simulink model "Vex2022Modle"  (R2022b)
settings: Solver=FixedStepAuto  StartTime=0.0  StopTime=inf  RelTol=1e-3  EnableMultiTasking=on
libraries: vexarmcortexlib x16, RoboticsPlayground x1
settings Model: Creator=carol  LastModifiedBy=carol
settings DataIOCC: LimitDataPoints=on  SignalLoggingSaveFormat=ModelDataLogs  ReturnWorkspaceOutputs=off
settings OptimizationCC: ExpressionDepthLimit=2147483647  LifeSpan=Inf  MaxStackSize=64  EfficientTunableParamExpr=on
settings DebuggingCC: UnderspecifiedInitializationDetection=Classic  MergeDetectMultiDrivingBlocksExec=none  InheritedTsInSrcMsg=none  FcnCallInpInsideContextMsg=warning  StateNameClashWarn=warning  SFUnexpectedBacktrackingDiag=warning  SFNoUnconditionalDefaultTransitionDiag=warning  SFExecutionAtInitializationDiag=none  SFMachineParentedDataDiag=warning  ArithmeticOperatorsInVariantConditions=warning
settings HardwareCC: ProdBitPerPointer=32  ProdBitPerSizeT=32  ProdBitPerPtrDiffT=32  ProdLargestAtomicInteger=Long  ProdLargestAtomicFloat=Double  ProdIntDivRoundTo=Undefined  ProdWordSize=32  ProdHWDeviceType=ARM Compatible->ARM Cortex
settings ModelReferenceCC: EnableRefExpFcnMdlSchedulingChecks=on  PropagateSignalLabelsOutOfModel=off
settings SFSimCC: MATLABDynamicMemAlloc=off  CustomCodeUndefinedFunction=UseInterfaceOnly
settings RTWCC: Description=Embedded Coder  SystemTargetFile=ert.tlc  HardwareBoard=ARM Cortex-based VEX Microcontroller  TemplateMakefile=ert_default_tmf  Toolchain=GNU Tools for VEX ARM Cortex
settings CodeAppCC: IgnoreCustomStorageClasses=off  CustomSymbolStrType=$N$R$M  StateflowObjectComments=on  InternalIdentifier=Classic
settings ERTTargetCC: CodeReplacementLibrary=GCC ARM Cortex-M3  MultiwordLength=2048  ConvertIfToSwitch=off  SuppressUnreachableDefaultCases=off

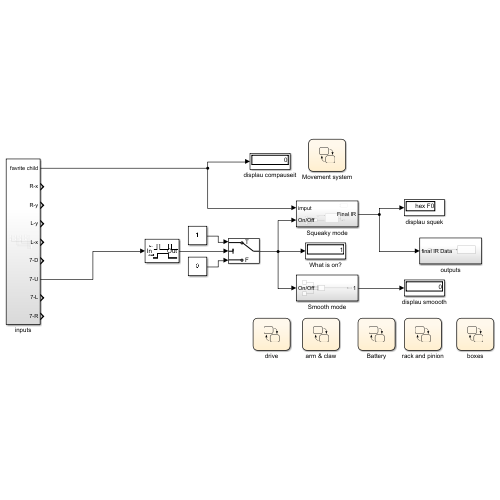
[thumbnail: Simulink's stored preview of the top-level diagram]
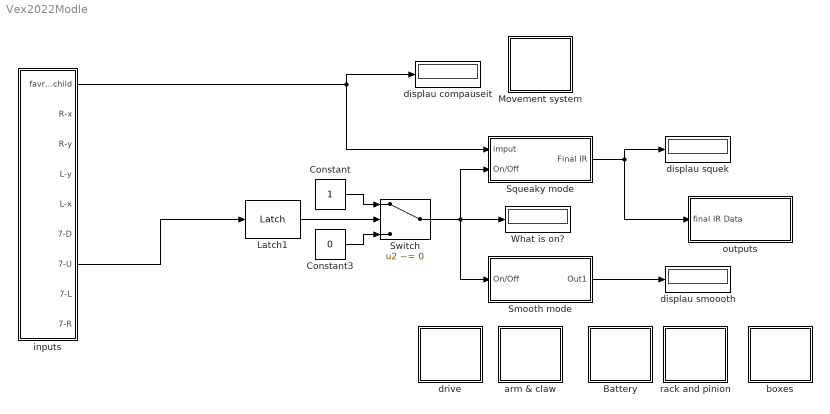
== system Vex2022Modle ==
  Battery : Stateflow chart  TreatAsAtomicUnit=on
  Constant : Constant
  Constant3 : Constant  Value=0
  Latch1 : RoboticsPlayground/Utilities and Hardware/Latch  SystemSampleTime=-1  VariantActivationTime=update diagram  Latency=0  AutoFrameSizeCalculation=off
      settings: SourceProductName=Robotics Playground
  Movement system : Stateflow chart  TreatAsAtomicUnit=on
  Smooth mode : Subsystem
  Squeaky mode : Subsystem
  Switch : Switch  Criteria=u2 ~= 0  SaturateOnIntegerOverflow=off  InputSameDT=off
  What is on? : Display
  arm & claw : Stateflow chart  TreatAsAtomicUnit=on
  boxes : Stateflow chart  TreatAsAtomicUnit=on
  displau compauseit : Display
  displau smoooth : Display
  displau squek : Display
      settings: Format=hex (Stored Integer)
  drive : Stateflow chart  TreatAsAtomicUnit=on
  inputs : Subsystem
  outputs : Subsystem
  rack and pinion : Stateflow chart  TreatAsAtomicUnit=on
  wires:
  Switch/1 -> What is on?/1, Smooth mode/1(On/Off), Squeaky mode/2(On/Off)
  Constant3/1 -> Switch/3
  Latch1/1 -> Switch/2
  inputs/1(favrite child) -> Squeaky mode/1(imput), displau compauseit/1
  inputs/7(7-U) -> Latch1/1
  Squeaky mode/1(Final IR) -> outputs/1(final IR Data), displau squek/1
  Constant/1 -> Switch/1
  Smooth mode/1(Out1) -> displau smoooth/1

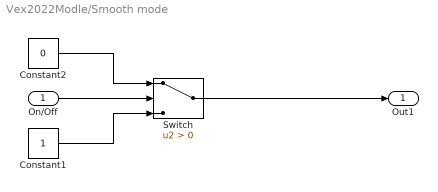
== system Vex2022Modle/Smooth mode ==
  On/Off : Inport
  Constant1 : Constant
  Constant2 : Constant  Value=0
  Switch : Switch  Criteria=u2 > Threshold  SaturateOnIntegerOverflow=off  InputSameDT=off
  Out1 : Outport
  wires:
  Switch/1 -> Out1/1
  Constant2/1 -> Switch/1
  On/Off/1 -> Switch/2
  Constant1/1 -> Switch/3

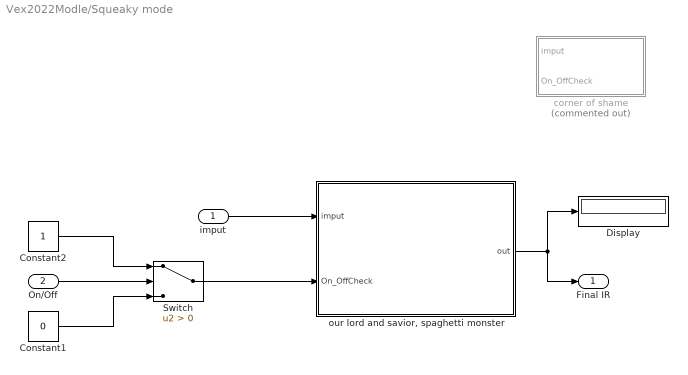
== system Vex2022Modle/Squeaky mode ==
  imput : Inport
  On/Off : Inport  Port=2
  Constant1 : Constant  Value=0
  Constant2 : Constant
  Display : Display
  Switch : Switch  Criteria=u2 > Threshold  SaturateOnIntegerOverflow=off  InputSameDT=off
  corner of shame : Stateflow chart  Commented=on  TreatAsAtomicUnit=on
  "our lord and savior, spaghetti monster" : Stateflow chart  TreatAsAtomicUnit=on
  Final IR : Outport
  wires:
  "our lord and savior, spaghetti monster"/1(out) -> Display/1, Final IR/1
  On/Off/1 -> Switch/2
  Constant1/1 -> Switch/3
  Constant2/1 -> Switch/1
  Switch/1 -> "our lord and savior, spaghetti monster"/2(On_OffCheck)
  imput/1 -> "our lord and savior, spaghetti monster"/1(imput)

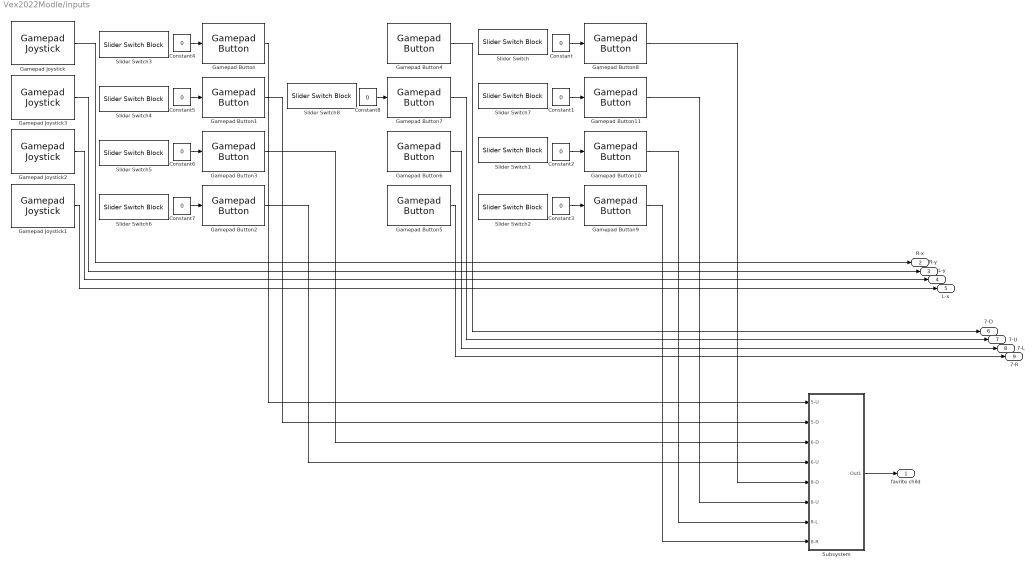
== system Vex2022Modle/inputs ==
  Constant{,1..8} (9 alike) : Constant  Value=0
  Gamepad Button : vexarmcortexlib/Gamepad/Gamepad Button  joystick=1  chan=5  button56=Up  button78=Down  SimulationIn=on  SampleTime=0.02
  Gamepad Button1 : vexarmcortexlib/Gamepad/Gamepad Button  joystick=1  chan=5  button56=Down  button78=Down  SimulationIn=on  SampleTime=0.02
  Gamepad Button10 : vexarmcortexlib/Gamepad/Gamepad Button  joystick=1  chan=8  button56=Up  button78=Left  SimulationIn=on  SampleTime=0.02
  Gamepad Button11 : vexarmcortexlib/Gamepad/Gamepad Button  joystick=1  chan=8  button56=Up  button78=Up  SimulationIn=on  SampleTime=0.02
  Gamepad Button2 : vexarmcortexlib/Gamepad/Gamepad Button  joystick=1  chan=6  button56=Up  button78=Down  SimulationIn=on  SampleTime=0.02
  Gamepad Button3 : vexarmcortexlib/Gamepad/Gamepad Button  joystick=1  chan=6  button56=Down  button78=Down  SimulationIn=on  SampleTime=0.02
  Gamepad Button4 : vexarmcortexlib/Gamepad/Gamepad Button  joystick=1  chan=7  button56=Up  button78=Down  SimulationIn=off  SampleTime=0.02
  Gamepad Button5 : vexarmcortexlib/Gamepad/Gamepad Button  joystick=1  chan=7  button56=Up  button78=Right  SimulationIn=off  SampleTime=0.02
  Gamepad Button6 : vexarmcortexlib/Gamepad/Gamepad Button  joystick=1  chan=7  button56=Up  button78=Left  SimulationIn=off  SampleTime=0.02
  Gamepad Button7 : vexarmcortexlib/Gamepad/Gamepad Button  joystick=1  chan=7  button56=Up  button78=Up  SimulationIn=on  SampleTime=0.02
  Gamepad Button8 : vexarmcortexlib/Gamepad/Gamepad Button  joystick=1  chan=8  button56=Up  button78=Down  SimulationIn=on  SampleTime=0.02
  Gamepad Button9 : vexarmcortexlib/Gamepad/Gamepad Button  joystick=1  chan=8  button56=Up  button78=Right  SimulationIn=on  SampleTime=0.02
  Gamepad Joystick : vexarmcortexlib/Gamepad/Gamepad Joystick  joystick=1  chan=1  SimulationIn=off  SampleTime=0.02
  Gamepad Joystick1 : vexarmcortexlib/Gamepad/Gamepad Joystick  joystick=1  chan=4  SimulationIn=off  SampleTime=0.02
  Gamepad Joystick2 : vexarmcortexlib/Gamepad/Gamepad Joystick  joystick=1  chan=3  SimulationIn=off  SampleTime=0.02
  Gamepad Joystick3 : vexarmcortexlib/Gamepad/Gamepad Joystick  joystick=1  chan=2  SimulationIn=off  SampleTime=0.02
  Slider Switch{,1..8} (9 alike) : SliderSwitchBlock
      settings: Values={{'Off', 'On'}, [0 1]}
  Subsystem : Subsystem
  favrite child : Outport
  R-x : Outport  Port=2
  R-y : Outport  Port=3
  L-y : Outport  Port=4
  L-x : Outport  Port=5
  7-D : Outport  Port=6
  7-U : Outport  Port=7
  7-L : Outport  Port=8
  7-R : Outport  Port=9
  wires:
  Gamepad Joystick/1 -> R-x/1
  Gamepad Joystick3/1 -> R-y/1
  Gamepad Joystick2/1 -> L-y/1
  Gamepad Joystick1/1 -> L-x/1
  Gamepad Button4/1 -> 7-D/1
  Gamepad Button7/1 -> 7-U/1
  Gamepad Button6/1 -> 7-L/1
  Gamepad Button5/1 -> 7-R/1
  Constant/1 -> Gamepad Button8/1
  Constant1/1 -> Gamepad Button11/1
  Constant2/1 -> Gamepad Button10/1
  Constant3/1 -> Gamepad Button9/1
  Constant4/1 -> Gamepad Button/1
  Constant5/1 -> Gamepad Button1/1
  Constant7/1 -> Gamepad Button2/1
  Constant6/1 -> Gamepad Button3/1
  Constant8/1 -> Gamepad Button7/1
  Gamepad Button/1 -> Subsystem/1(5-U)
  Gamepad Button1/1 -> Subsystem/2(5-D)
  Gamepad Button3/1 -> Subsystem/3(6-D)
  Gamepad Button2/1 -> Subsystem/4(6-U)
  Gamepad Button8/1 -> Subsystem/5(8-D)
  Gamepad Button11/1 -> Subsystem/6(8-U)
  Gamepad Button10/1 -> Subsystem/7(8-L)
  Gamepad Button9/1 -> Subsystem/8(8-R)
  Subsystem/1(Out1) -> favrite child/1

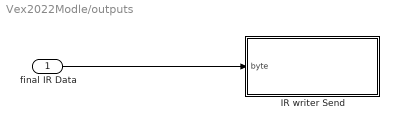
== system Vex2022Modle/outputs ==
  final IR Data : Inport
  IR writer Send : Subsystem
  wires:
  final IR Data/1 -> IR writer Send/1(byte)

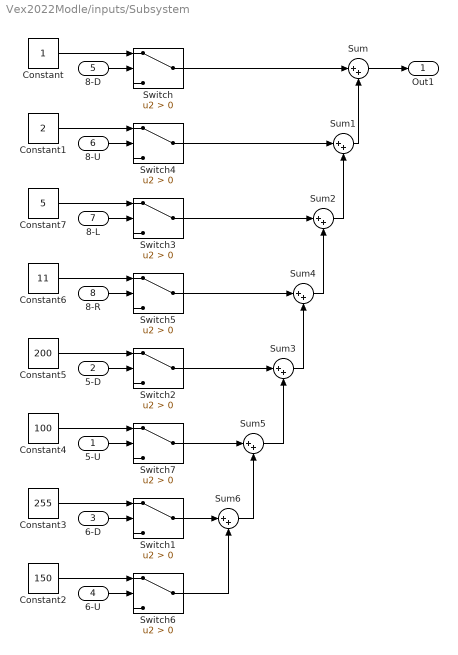
== system Vex2022Modle/inputs/Subsystem ==
  5-U : Inport
  5-D : Inport  Port=2
  6-D : Inport  Port=3
  6-U : Inport  Port=4
  8-D : Inport  Port=5
  8-U : Inport  Port=6
  8-L : Inport  Port=7
  8-R : Inport  Port=8
  Constant : Constant
  Constant1 : Constant  Value=2
  Constant2 : Constant  Value=150
  Constant3 : Constant  Value=255
  Constant4 : Constant  Value=100
  Constant5 : Constant  Value=200
  Constant6 : Constant  Value=11
  Constant7 : Constant  Value=5
  Sum{,1..6} (7 alike) : Sum  Inputs=|++
  Switch{,1..7} (8 alike) : Switch  Criteria=u2 > Threshold  SaturateOnIntegerOverflow=off  InputSameDT=off
  Out1 : Outport
  wires:
  8-D/1 -> Switch/2
  Sum/1 -> Out1/1
  Switch4/1 -> Sum1/1
  Sum1/1 -> Sum/2
  Switch3/1 -> Sum2/1
  Sum2/1 -> Sum1/2
  Switch5/1 -> Sum4/1
  Switch6/1 -> Sum6/2
  Switch1/1 -> Sum6/1
  Switch7/1 -> Sum5/1
  Switch2/1 -> Sum3/1
  Sum4/1 -> Sum2/2
  Sum3/1 -> Sum4/2
  Sum5/1 -> Sum3/2
  Sum6/1 -> Sum5/2
  Switch/1 -> Sum/1
  8-U/1 -> Switch4/2
  8-L/1 -> Switch3/2
  6-U/1 -> Switch6/2
  6-D/1 -> Switch1/2
  5-U/1 -> Switch7/2
  5-D/1 -> Switch2/2
  8-R/1 -> Switch5/2
  Constant/1 -> Switch/1
  Constant1/1 -> Switch4/1
  Constant7/1 -> Switch3/1
  Constant5/1 -> Switch2/1
  Constant6/1 -> Switch5/1
  Constant2/1 -> Switch6/1
  Constant4/1 -> Switch7/1
  Constant3/1 -> Switch1/1

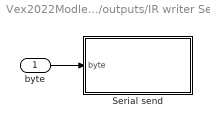
== system Vex2022Modle/outputs/IR writer Send ==
  byte : Inport  OutDataTypeStr=uint8  PortDimensions=[1 1]
  Serial send : MATLAB Function  TreatAsAtomicUnit=on
  wires:
  byte/1 -> Serial send/1(byte)

== stateflow chart Vex2022Modle/arm & claw ==

== stateflow chart Vex2022Modle/Battery ==

== stateflow chart Vex2022Modle/rack and pinion ==

== stateflow chart Vex2022Modle/boxes ==

== stateflow chart Vex2022Modle/Squeaky mode/corner of shame ==
  state Test
    finalData = 0xF0;
    imput = 0;
  state CenterD
    finalData  = 0x66;
    imput = 0;
  state Initialize
    finalData =0x00;
  state CenterR
    finalData = 0xCC;
    imput = 0;
  state CenterL
    finalData = 0x5A;
    imput = 0;
  Initialize -> Test [order 1] : [imput == 1]
  Test -> Initialize
  Initialize -> CenterD [order 2] : [imput == 2]
  CenterD -> Initialize
  (default) -> Initialize : {On_OffCheck == 1}
  CenterR -> Initialize
  Initialize -> CenterL [order 3] : [imput == 4]
  CenterL -> Initialize
  Initialize -> CenterR [order 4] : [imput == 3]
  data: imput input; On_OffCheck input

== stateflow chart Vex2022Modle/Squeaky mode/our lord and savior, spaghetti monster ==
  state Speed Adjustments [group]
    state nyoomHigh
      entry:
      out = 0xC3;
    state nyoomLow
      entry:
      out = 0x99;
    state nyoomMed
      entry:
      out = 0xA5;
  state onOff
  state Squeaky Movements [group]
    state lift_2
      entry:
      out = 0x5A;
    state drive_2
      entry:
      out = 0x3C;
    state rotate_2
      entry:
      out = 0x33;
  state irTestDefault
    entry:
    out = 0xF0;
  state Rotational Adjustments [group]
    state spinspinHigh
      entry:
      out = 0x0F;
    state spinspinLow
      entry:
      out = 0x69;
    state spinspinMed
      entry:
      out = 0x96;
  (default) -> onOff
  irTestDefault -> nyoomHigh [order 4] : [imput == 100]
  nyoomHigh -> irTestDefault : [imput ~= 100]
  onOff -> irTestDefault : [On_OffCheck == 1]
  irTestDefault -> lift_2 [order 1] : [imput == 5]
  irTestDefault -> nyoomLow [order 7] : [imput == 200]
  lift_2 -> irTestDefault : [imput ~= 5]
  nyoomLow -> irTestDefault : [imput ~= 200]
  irTestDefault -> nyoomMed [order 8] : [imput==300]
  nyoomMed -> irTestDefault : [imput ~= 300]
  spinspinHigh -> irTestDefault : [imput ~= 150]
  irTestDefault -> drive_2 [order 2] : [imput == 1]
  drive_2 -> irTestDefault : [imput ~=1]
  irTestDefault -> spinspinHigh [order 6] : [imput == 150]
  irTestDefault -> spinspinLow [order 5] : [imput == 255]
  spinspinLow -> irTestDefault : [imput ~= 250]
  irTestDefault -> spinspinMed [order 9] : [imput == 405]
  spinspinMed -> irTestDefault : [imput ~= 405]
  rotate_2 -> irTestDefault : [imput ~= 11]
  irTestDefault -> rotate_2 [order 3] : [imput == 11]
  data: imput input; out output; On_OffCheck input

== stateflow chart Vex2022Modle/Movement system ==

== matlab function Vex2022Modle/outputs/IR writer Send/Serial send ==
  data: byte input
function fcn(byte)
% Serial send single byte
%#codegen

% Config
port = 'uart1';
baud = uint32(9600);

persistent isFirstRun

if coder.target('Rtw')
    coder.cinclude('API.h');
    coder.cinclude('string.h');
    file = coder.opaque('FILE *', port,'HeaderFile','API.h');

    if isempty(isFirstRun)
        % first time setup
        isFirstRun = false;

        flags = coder.opaque('uint16', 'SERIAL_8N1');
        coder.ceval('usartInit', file, baud, flags);
    end

    coder.ceval('fputc', byte, file);

end

end

== stateflow chart Vex2022Modle/drive ==
